simulink model "lqr_controller_of_rocket_simulink_model"  (R2020a)
settings: Solver=FixedStepAuto  StartTime=0.0  StopTime=.01  FixedStep=.000001  RelTol=1e-3
values from neighbouring files (symbols this model uses):
  g = 9.81    [calculate_LQR_gains.m]
  I_sp = 2770    [calculate_LQR_gains.m]
  L = l    (= 70)    [calculate_LQR_gains.m]
  m0 = 34284    [calculate_LQR_gains.m]
  mf = 549054    [calculate_LQR_gains.m]
  r = 3.66/2    (= 1.83)    [calculate_LQR_gains.m]
  x0 = [o, o, o, 0, o, o, 90, 15, -90, ((m0+mf)/2), o]    [calculate_LQR_gains.m]
undefined symbols (not defined in the file or in its folder): K
libraries: modelsimlib x1
settings Model: Creator=paull  LastModifiedBy=SSS
settings DataIOCC: ReturnWorkspaceOutputs=off
settings DebuggingCC: ArithmeticOperatorsInVariantConditions=warning
settings SFSimCC: SimUseLocalCustomCode=off  CustomCodeUndefinedFunction=UseInterfaceOnly
settings RTWCC: RTWUseLocalCustomCode=off

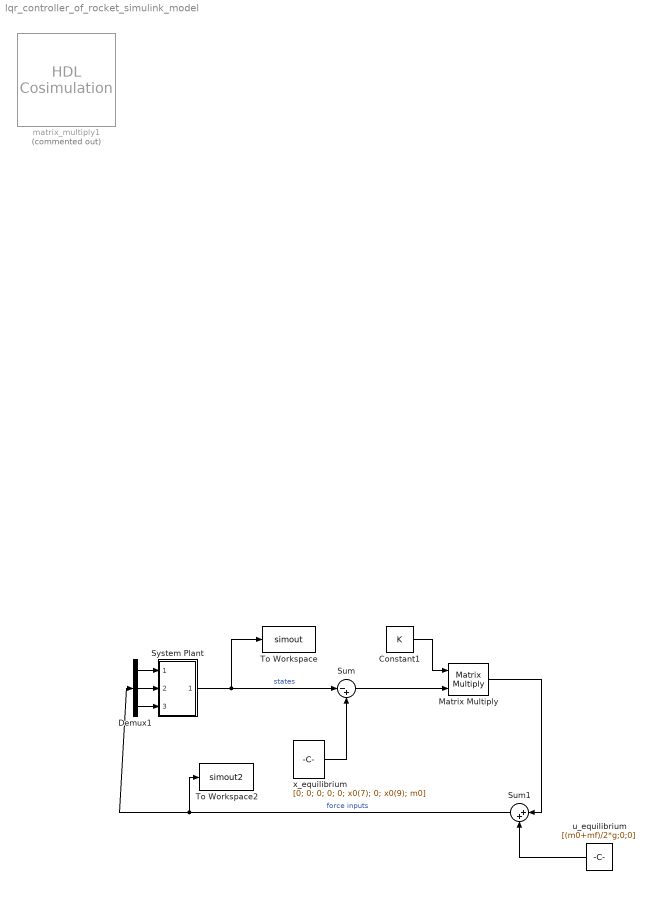
== system lqr_controller_of_rocket_simulink_model ==
  Constant1 : Constant  Value=K
  Demux1 : Demux  Outputs=3
  Matrix Multiply : Product  Multiplication=Matrix(*)
  Sum : Sum  Inputs=|-+
  Sum1 : Sum  Inputs=|++
  System Plant : Subsystem
  To Workspace : ToWorkspace  VariableName=simout  SaveFormat=Structure With Time  SampleTime=-1
  To Workspace2 : ToWorkspace  VariableName=simout2  SaveFormat=Structure With Time  SampleTime=-1
  matrix_multiply1 : modelsimlib/HDL Cosimulation  Commented=on  PortPaths=/matrix_multiply/input_gains_matrix;/matrix_multiply/input_states_matrix;/matrix_multiply/sample_time;/matrix_multiply/output_matrix;/matrix_multiply/output_valid  PortModes=[1 1 1 2 2 ]  PortTimes=[-1,-1,-1,.00000000000001,.00000000000001]  PortSigns=[-1 -1 -1 -1 -1 ]  PortFracLengths=[0,0,0,0,0]  CommLocal=on  CommSharedMemory=on  CommPortNumber=4449  CommShowInfo=on  ClockModes=[]  ClockTimes=[]  TclPreSimCommand=|  TclPostSimCommand=|  TimingMode=ns  TimingScaleFactor=1  idxCellArray={'UNUSED_VAR'}  CosimBypass=Full Simulation  AllowDirectFeedthrough=on  ProductName=EDA Simulator Link MQ  RunAutoTimescale=off  HdlClocks=/matrix_multiply/clock 10 ns;  PreRunTime=10  PreRunTimeUnit=ns
      TclPreSimCommand=|
      | force /matrix_multiply/clock 0 0 ns, 1 5 ns -repeat 10 ns;
      | force /matrix_multiply/reset 1 0 ns, 0 8 ns;
      TclPostSimCommand=|
      | noforce /matrix_multiply/clock;
      | noforce /matrix_multiply/reset;
      | puts "done";
      settings: SourceProductBaseCode=ES
  u_equilibrium : Constant  Value=[(m0+mf)/2*g;0;0]
  x_equilibrium : Constant  Value=[0; 0; 0; 0; 0; x0(7); 0; x0(9); m0]
  wires:
  Constant1/1 -> Matrix Multiply/1
  Demux1/1 -> System Plant/1(In1)
  Demux1/2 -> System Plant/2(In2)
  Demux1/3 -> System Plant/3(In3)
  System Plant/1(Out2) -> To Workspace/1, Sum/1  "states"
  x_equilibrium/1 -> Sum/2
  Sum/1 -> Matrix Multiply/2
  Matrix Multiply/1 -> Sum1/1
  Sum1/1 -> To Workspace2/1, Demux1/1  "force inputs"
  u_equilibrium/1 -> Sum1/2

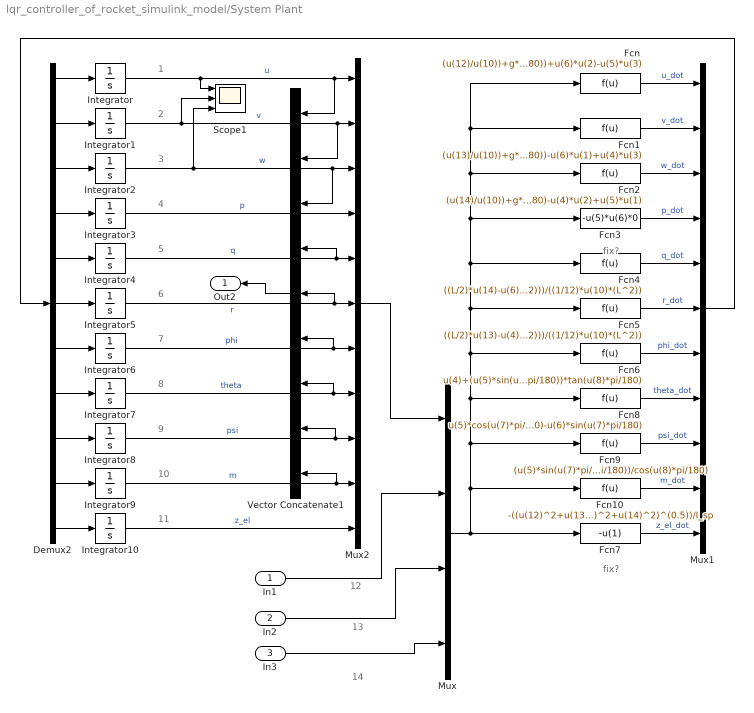
== system lqr_controller_of_rocket_simulink_model/System Plant ==
  note: 14
  note: fix?
  note: 2
  note: 3
  note: 4
  note: 5
  note: 8
  note: 6
  note: 7
  note: 9
  note: 11
  note: 10
  note: 1
  note: fix?
  note: 12
  note: 13
  In1 : Inport
  In2 : Inport  Port=2
  In3 : Inport  Port=3
  Demux2 : Demux  Outputs=11
  Fcn : Fcn  Expr=(u(12)/u(10))+g*(cos(u(7)*pi/180)*sin(u(8)*pi/180)*cos(u(9)*pi/180)+sin(u(7)*pi/180)*sin(u(9)*pi/180))+u(6)*u(2)-u(5)*u(3)
  Fcn1 : Fcn  Expr=(u(13)/u(10))+g*(cos(u(7)*pi/180)*sin(u(8)*pi/180)*cos(u(9)*pi/180)-sin(u(7)*pi/180)*cos(u(9)*pi/180))-u(6)*u(1)+u(4)*u(3)
  Fcn10 : Fcn  Expr=-((u(12)^2+u(13)^2+u(14)^2)^(0.5))/I_sp
  Fcn2 : Fcn  Expr=(u(14)/u(10))+g*cos(u(7)*pi/180)*cos(u(8)*pi/180)-u(4)*u(2)+u(5)*u(1)
  Fcn3 : Fcn  Expr=-u(5)*u(6)*0
  Fcn4 : Fcn  Expr=((L/2)*u(14)-u(6)*u(4)*(0.5*u(10)*(r^2)-(1/12)*u(10)*(L^2)))/((1/12)*u(10)*(L^2))
  Fcn5 : Fcn  Expr=((L/2)*u(13)-u(4)*u(5)*((1/12)*u(10)*(L^2)-0.5*u(10)*(r^2)))/((1/12)*u(10)*(L^2))
  Fcn6 : Fcn  Expr=u(4)+(u(5)*sin(u(7)*pi/180)+u(6)*cos(u(7)*pi/180))*tan(u(8)*pi/180)
  Fcn7 : Fcn  Expr=-u(1)
  Fcn8 : Fcn  Expr=u(5)*cos(u(7)*pi/180)-u(6)*sin(u(7)*pi/180)
  Fcn9 : Fcn  Expr=(u(5)*sin(u(7)*pi/180)+u(6)*cos(u(7)*pi/180))/cos(u(8)*pi/180)
  Integrator : Integrator  InitialCondition=x0(1)
  Integrator1 : Integrator  InitialCondition=x0(2)
  Integrator10 : Integrator  InitialCondition=x0(11)
  Integrator2 : Integrator  InitialCondition=x0(3)
  Integrator3 : Integrator  InitialCondition=x0(4)
  Integrator4 : Integrator  InitialCondition=x0(5)
  Integrator5 : Integrator  InitialCondition=x0(6)
  Integrator6 : Integrator  InitialCondition=x0(7)
  Integrator7 : Integrator  InitialCondition=x0(8)
  Integrator8 : Integrator  InitialCondition=x0(9)
  Integrator9 : Integrator  InitialCondition=x0(10)
  Mux : Mux
  Mux1 : Mux  Inputs=11
  Mux2 : Mux  Inputs=11
  Scope1 : Scope  NumInputPorts=3
  Vector Concatenate1 : Concatenate  NumInputs=9
  Out2 : Outport  VectorParamsAs1DForOutWhenUnconnected=off
  wires:
  Mux/1 -> Fcn6/1, Fcn5/1, Fcn4/1, Fcn3/1, Fcn2/1, Fcn1/1, Fcn/1, Fcn8/1, Fcn9/1, Fcn10/1, Fcn7/1
  Demux2/5 -> Integrator4/1
  Demux2/1 -> Integrator/1
  Demux2/8 -> Integrator7/1
  Integrator10/1 -> Mux2/11  "z_el"
  Vector Concatenate1/1 -> Out2/1
  Integrator5/1 -> Vector Concatenate1/5, Mux2/6  "r"
  Demux2/3 -> Integrator2/1
  Mux2/1 -> Mux/1
  Integrator3/1 -> Mux2/4  "p"
  Integrator4/1 -> Vector Concatenate1/4, Mux2/5  "q"
  Demux2/11 -> Integrator10/1
  Integrator8/1 -> Vector Concatenate1/8, Mux2/9  "psi"
  Integrator9/1 -> Vector Concatenate1/9, Mux2/10  "m"
  In2/1 -> Mux/3
  Demux2/10 -> Integrator9/1
  Integrator2/1 -> Vector Concatenate1/3, Mux2/3, Scope1/3  "w"
  Mux1/1 -> Demux2/1
  Demux2/4 -> Integrator3/1
  Integrator/1 -> Vector Concatenate1/1, Mux2/1, Scope1/1  "u"
  Fcn4/1 -> Mux1/5  "q_dot"
  Demux2/7 -> Integrator6/1
  In1/1 -> Mux/2
  Demux2/2 -> Integrator1/1
  Integrator1/1 -> Vector Concatenate1/2, Mux2/2, Scope1/2  "v"
  Fcn7/1 -> Mux1/11  "z_el_dot"
  Fcn1/1 -> Mux1/2  "v_dot"
  Fcn2/1 -> Mux1/3  "w_dot"
  Fcn5/1 -> Mux1/6  "r_dot"
  Fcn3/1 -> Mux1/4  "p_dot"
  Demux2/9 -> Integrator8/1
  Fcn8/1 -> Mux1/8  "theta_dot"
  Fcn6/1 -> Mux1/7  "phi_dot"
  Demux2/6 -> Integrator5/1
  Fcn9/1 -> Mux1/9  "psi_dot"
  Fcn/1 -> Mux1/1  "u_dot"
  Integrator6/1 -> Vector Concatenate1/6, Mux2/7  "phi"
  Integrator7/1 -> Vector Concatenate1/7, Mux2/8  "theta"
  Fcn10/1 -> Mux1/10  "m_dot"
  In3/1 -> Mux/4
